simulink model "DCmotTime"  (Simulink 6.1)
settings: Solver=FixedStepDiscrete  SolverMode=SingleTasking  StartTime=0.0  StopTime=inf  FixedStep=0.001  RelTol=1e-3
undefined symbols (not defined in the file): simget
libraries: qctools x2
settings Model: LastModifiedBy=m133768  ExtModeArmWhenConnect=off  BufferReuse=off
settings ConfigSet: SimulationMode=external
settings OptimizationCC: BooleanDataType=off  OptimizeBlockIOStorage=off  BufferReuse=off  ExpressionFolding=off  LocalBlockOutputs=off
settings DebuggingCC: SolverPrmCheckMsg=warning
settings RTWCC: SystemTargetFile=wincon.tlc  MakeCommand=make_wc  TemplateMakefile=wc_default_tmf  Description=WinCon Target  ProcessScript=wincon_make_rtw_hook
settings STFCustomTargetCC: TargetFcnLib=ansi_tfl_tmw.mat  GenFloatMathFcnCalls=ANSI_C  ModelReferenceCompliant=off  SystemTargetFile=wincon.tlc
settings GRTTargetCC: ModelReferenceCompliant=off  MatFileLogging=off  ExtMode=on  ExtModeTransport=2  ExtModeMexFile=wc_comm
settings CustomProperty: Value=on

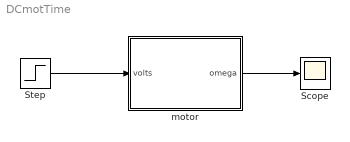
== system DCmotTime ==
  Scope : Scope
  Step : Step  Time=2  Before=3  After=23.89  SampleTime=0
  motor : Subsystem
  wires:
  Step/1 -> motor/1(volts)
  motor/1(omega) -> Scope/1

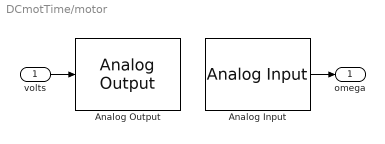
== system DCmotTime/motor ==
  volts : Inport  Port=1  LatchInput=off
  Analog Input : qctools/Quanser Consulting MultiQ-PCI Series/Analog Input  boardNumber=0  channels=2  ranges=10  sampleTime=simget(bdroot,'FixedStep')  simulationInput=off
  Analog Output : qctools/Quanser Consulting MultiQ-PCI Series/Analog Output  boardNumber=0  channels=0  initialOutputs=0  finalOutputs=0  sampleTime=-1  simulationOutput=off
  omega : Outport
  wires:
  Analog Input/1 -> omega/1
  volts/1 -> Analog Output/1
